simulink model "DroneModel"  (R2021b)
settings: Solver=VariableStepAuto  StartTime=0.0  StopTime=5  RelTol=1e-3
values from neighbouring files (symbols this model uses):
  g = 9.8    [testModel.m]
  Im = 0.0135^2*0.045/2    (= 4.100625e-06)    [testModel.m]
  Ip = (1.8*r)^2*0.015/12    (= 1.9845e-05)    [testModel.m]
  Ix = m/3*a^2/12+2*0.045*l^2    (= 0.00211347222222)    [testModel.m]
  Iy = m/3*a^2/12+4*0.045*l^2    (= 0.00413847222222)    [testModel.m]
  Iz = m/3*a^2/4+2*0.045*l^2    (= 0.00229041666667)    [testModel.m]
  J = 2.5*10^(-6)    (= 2.5e-06)    [testModel.m]
  Ke = ke    (= 0.0073)    [testModel.m]
  kf = ks*r^2*airDensity*Sblade/2    (= 1.57565625e-05)    [testModel.m]
  Km = kt    (= 0.0073)    [testModel.m]
  l = 0.15    [testModel.m]
  m = 0.65    [testModel.m]
  maxU = 11    [testModel.m]
  r = 0.07    [testModel.m]
  R = ra    (= 0.048)    [testModel.m]
  U1 = U1_arr(i)    [testModel.m]
  U2 = U2_arr(i)    [testModel.m]
  U3 = U3_arr(i)    [testModel.m]
  U4 = U4_arr(i)    [testModel.m]
settings Model: Creator=Degra  LastModifiedBy=Degra

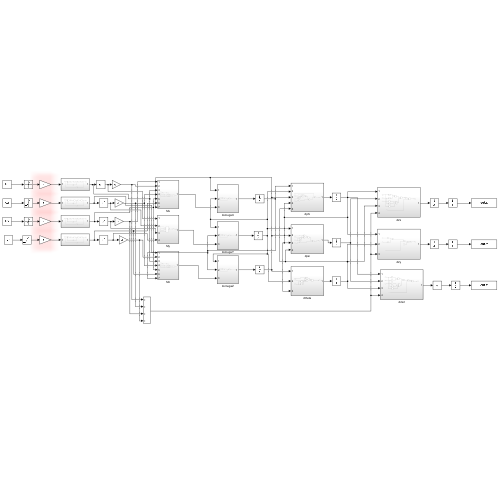
[thumbnail: Simulink's stored preview of the top-level diagram]
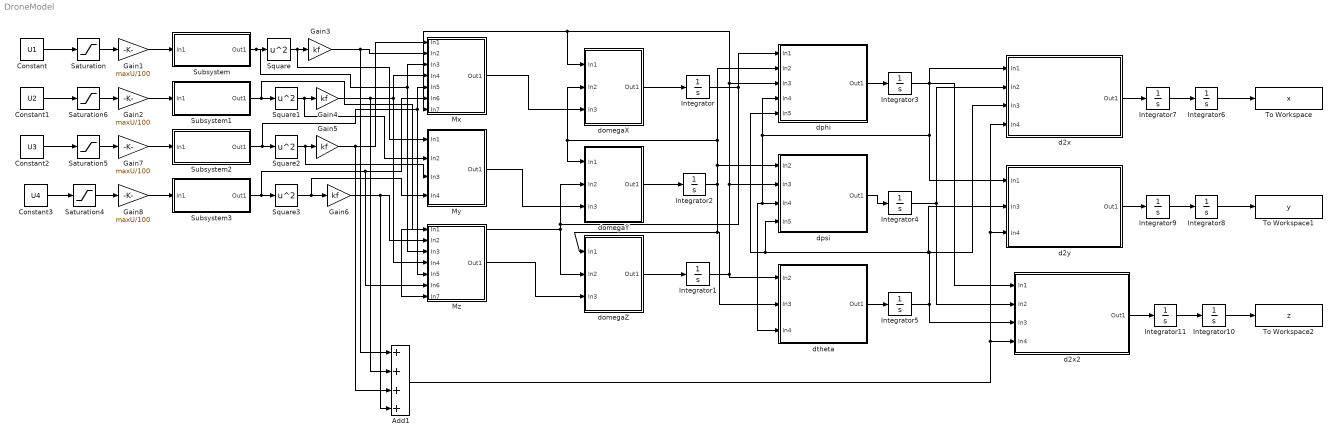
== system DroneModel ==
  Add1 : Sum  Inputs=++++
  Constant : Constant  Value=U1
  Constant1 : Constant  Value=U2
  Constant2 : Constant  Value=U3
  Constant3 : Constant  Value=U4
  Gain{1..2,7..8} (4 alike) : Gain  Gain=maxU/100
  Gain{3..6} (4 alike) : Gain  Gain=kf
  Integrator{,1..11} (12 alike) : Integrator
  Mx : Subsystem
  My : Subsystem
  Mz : Subsystem
  Saturation{,4..6} (4 alike) : Saturate  UpperLimit=100  LowerLimit=-100
  Square{,1..3} (4 alike) : Math  Operator=square  SaturateOnIntegerOverflow=on
  Subsystem : Subsystem
  Subsystem1 : Subsystem
  Subsystem2 : Subsystem
  Subsystem3 : Subsystem
  To Workspace : ToWorkspace  VariableName=x  SaveFormat=Timeseries  SampleTime=-1
  To Workspace1 : ToWorkspace  VariableName=y  SaveFormat=Timeseries  SampleTime=-1
  To Workspace2 : ToWorkspace  VariableName=z  SaveFormat=Timeseries  SampleTime=-1
  d2x : Subsystem
  d2x2 : Subsystem
  d2y : Subsystem
  domegaX : Subsystem
  domegaY : Subsystem
  domegaZ : Subsystem
  dphi : Subsystem
  dpsi : Subsystem
  dtheta : Subsystem
  wires:
  Subsystem/1(Out1) -> Mz/3(In3), Mx/3(In3), Square/1
  Square/1 -> My/1(In1), Gain3/1
  Subsystem1/1(Out1) -> Add1/2, Mz/4(In4), Mx/4(In4), Square1/1
  Square1/1 -> My/2(In2), Gain4/1
  Square2/1 -> My/3(In3), Gain5/1
  Subsystem3/1(Out1) -> Mz/6(In6), Mx/6(In6), Square3/1
  Square3/1 -> My/4(In4), Gain6/1
  Gain5/1 -> Add1/3, Mx/1(In1)
  Gain3/1 -> Add1/1, Mx/2(In2)
  Gain4/1 -> Mz/1(In1)
  Gain6/1 -> Add1/4, Mz/2(In2)
  Subsystem2/1(Out1) -> Mz/5(In5), Mx/5(In5), Square2/1
  Mx/1(Out1) -> domegaX/3(In3)
  domegaX/1(Out1) -> Integrator/1
  Integrator/1 -> domegaZ/2(In2), Mz/7(In7), domegaY/2(In2), dphi/1(In1)
  domegaZ/1(Out1) -> Integrator1/1
  Integrator1/1 -> dtheta/1(In2), dphi/3(In3), domegaX/1(In1), Mx/7(In7), dpsi/2(In3)
  Mz/1(Out1) -> domegaZ/3(In3)
  My/1(Out1) -> domegaY/3(In3)
  domegaY/1(Out1) -> Integrator2/1
  Integrator2/1 -> dphi/2(In2), domegaY/1(In1), domegaX/2(In2), dpsi/1(In2), domegaZ/1(In1), dtheta/2(In3)
  dpsi/1(Out1) -> Integrator4/1
  dphi/1(Out1) -> Integrator3/1
  Integrator3/1 -> d2x2/1(In1), d2x/1(In1), d2y/1(In1), dtheta/3(In4), dpsi/3(In4), dphi/4(In4)
  dtheta/1(Out1) -> Integrator5/1
  Integrator5/1 -> d2x2/3(In3), d2x/3(In3), d2y/2(In3), dpsi/4(In5), dphi/5(In5)
  Integrator4/1 -> d2x2/2(In2), d2x/2(In2)
  Add1/1 -> d2x2/4(In4), d2y/3(In4), d2x/4(In4)
  d2x/1(Out1) -> Integrator7/1
  Integrator7/1 -> Integrator6/1
  Integrator9/1 -> Integrator8/1
  d2y/1(Out1) -> Integrator9/1
  Integrator11/1 -> Integrator10/1
  d2x2/1(Out1) -> Integrator11/1
  Integrator6/1 -> To Workspace/1
  Integrator8/1 -> To Workspace1/1
  Integrator10/1 -> To Workspace2/1
  Constant/1 -> Saturation/1
  Constant3/1 -> Saturation4/1
  Constant2/1 -> Saturation5/1
  Constant1/1 -> Saturation6/1
  Saturation/1 -> Gain1/1
  Saturation6/1 -> Gain2/1
  Saturation4/1 -> Gain8/1
  Gain1/1 -> Subsystem/1(In1)
  Gain8/1 -> Subsystem3/1(In1)
  Gain7/1 -> Subsystem2/1(In1)
  Gain2/1 -> Subsystem1/1(In1)
  Saturation5/1 -> Gain7/1

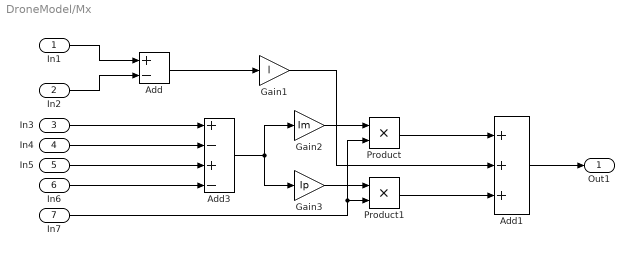
== system DroneModel/Mx ==
  In1 : Inport
  In2 : Inport  Port=2
  In3 : Inport  Port=3
  In4 : Inport  Port=4
  In5 : Inport  Port=5
  In6 : Inport  Port=6
  In7 : Inport  Port=7
  Add : Sum  Inputs=+-
  Add1 : Sum  Inputs=+++
  Add3 : Sum  Inputs=+-+-
  Gain1 : Gain  Gain=l
  Gain2 : Gain  Gain=Im
  Gain3 : Gain  Gain=Ip
  Product : Product
  Product1 : Product
  Out1 : Outport
  wires:
  In1/1 -> Add/1
  In2/1 -> Add/2
  In3/1 -> Add3/1
  In4/1 -> Add3/2
  In5/1 -> Add3/3
  In6/1 -> Add3/4
  Add/1 -> Gain1/1
  Add3/1 -> Gain3/1, Gain2/1
  Gain3/1 -> Product1/1
  Gain2/1 -> Product/1
  In7/1 -> Product1/2, Product/2
  Product1/1 -> Add1/3
  Product/1 -> Add1/1
  Gain1/1 -> Add1/2
  Add1/1 -> Out1/1

== system DroneModel/My ==
  In1 : Inport
  In2 : Inport  Port=2
  In3 : Inport  Port=3
  In4 : Inport  Port=4
  Add3 : Sum  Inputs=-+-+
  Gain3 : Gain  Gain=kf*r
  Out1 : Outport
  wires:
  Add3/1 -> Gain3/1
  In1/1 -> Add3/1
  In2/1 -> Add3/2
  In3/1 -> Add3/3
  In4/1 -> Add3/4
  Gain3/1 -> Out1/1

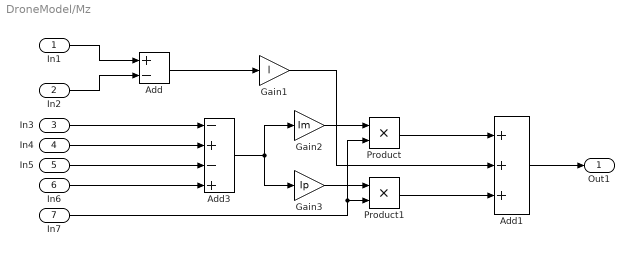
== system DroneModel/Mz ==
  In1 : Inport
  In2 : Inport  Port=2
  In3 : Inport  Port=3
  In4 : Inport  Port=4
  In5 : Inport  Port=5
  In6 : Inport  Port=6
  In7 : Inport  Port=7
  Add : Sum  Inputs=+-
  Add1 : Sum  Inputs=+++
  Add3 : Sum  Inputs=-+-+
  Gain1 : Gain  Gain=l
  Gain2 : Gain  Gain=Im
  Gain3 : Gain  Gain=Ip
  Product : Product
  Product1 : Product
  Out1 : Outport
  wires:
  In1/1 -> Add/1
  In2/1 -> Add/2
  In3/1 -> Add3/1
  In4/1 -> Add3/2
  In5/1 -> Add3/3
  In6/1 -> Add3/4
  Add/1 -> Gain1/1
  Add3/1 -> Gain3/1, Gain2/1
  Gain3/1 -> Product1/1
  Gain2/1 -> Product/1
  In7/1 -> Product1/2, Product/2
  Product1/1 -> Add1/3
  Product/1 -> Add1/1
  Gain1/1 -> Add1/2
  Add1/1 -> Out1/1

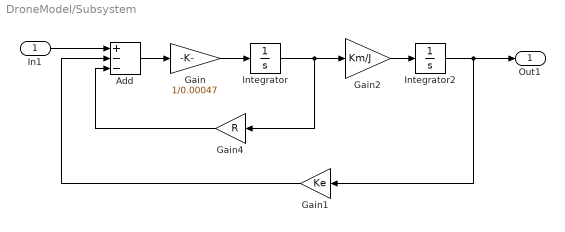
== system DroneModel/Subsystem ==
  In1 : Inport
  Add : Sum  Inputs=+--
  Gain : Gain  Gain=1/0.00047
  Gain1 : Gain  Gain=Ke
  Gain2 : Gain  Gain=Km/J
  Gain4 : Gain  Gain=R
  Integrator : Integrator
  Integrator2 : Integrator
  Out1 : Outport
  wires:
  In1/1 -> Add/1
  Gain4/1 -> Add/3
  Gain1/1 -> Add/2
  Integrator2/1 -> Out1/1, Gain1/1
  Integrator/1 -> Gain2/1, Gain4/1
  Gain2/1 -> Integrator2/1
  Add/1 -> Gain/1
  Gain/1 -> Integrator/1

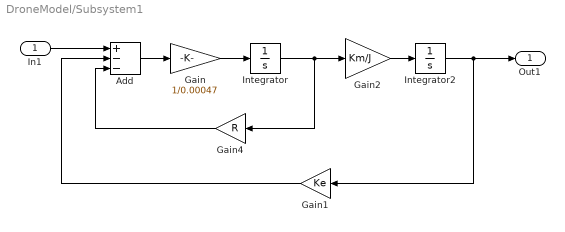
== system DroneModel/Subsystem1 ==
  In1 : Inport
  Add : Sum  Inputs=+--
  Gain : Gain  Gain=1/0.00047
  Gain1 : Gain  Gain=Ke
  Gain2 : Gain  Gain=Km/J
  Gain4 : Gain  Gain=R
  Integrator : Integrator
  Integrator2 : Integrator
  Out1 : Outport
  wires:
  In1/1 -> Add/1
  Gain4/1 -> Add/3
  Gain1/1 -> Add/2
  Integrator2/1 -> Out1/1, Gain1/1
  Integrator/1 -> Gain2/1, Gain4/1
  Gain2/1 -> Integrator2/1
  Add/1 -> Gain/1
  Gain/1 -> Integrator/1

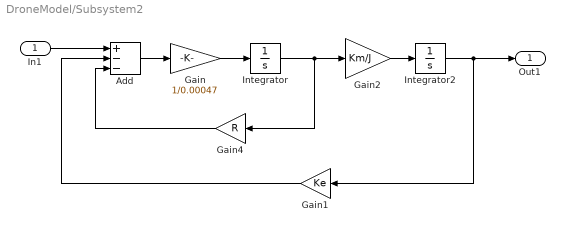
== system DroneModel/Subsystem2 ==
  In1 : Inport
  Add : Sum  Inputs=+--
  Gain : Gain  Gain=1/0.00047
  Gain1 : Gain  Gain=Ke
  Gain2 : Gain  Gain=Km/J
  Gain4 : Gain  Gain=R
  Integrator : Integrator
  Integrator2 : Integrator
  Out1 : Outport
  wires:
  In1/1 -> Add/1
  Gain4/1 -> Add/3
  Gain1/1 -> Add/2
  Integrator2/1 -> Out1/1, Gain1/1
  Integrator/1 -> Gain2/1, Gain4/1
  Gain2/1 -> Integrator2/1
  Add/1 -> Gain/1
  Gain/1 -> Integrator/1

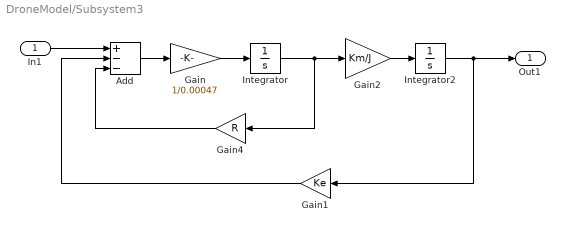
== system DroneModel/Subsystem3 ==
  In1 : Inport
  Add : Sum  Inputs=+--
  Gain : Gain  Gain=1/0.00047
  Gain1 : Gain  Gain=Ke
  Gain2 : Gain  Gain=Km/J
  Gain4 : Gain  Gain=R
  Integrator : Integrator
  Integrator2 : Integrator
  Out1 : Outport
  wires:
  In1/1 -> Add/1
  Gain4/1 -> Add/3
  Gain1/1 -> Add/2
  Integrator2/1 -> Out1/1, Gain1/1
  Integrator/1 -> Gain2/1, Gain4/1
  Gain2/1 -> Integrator2/1
  Add/1 -> Gain/1
  Gain/1 -> Integrator/1

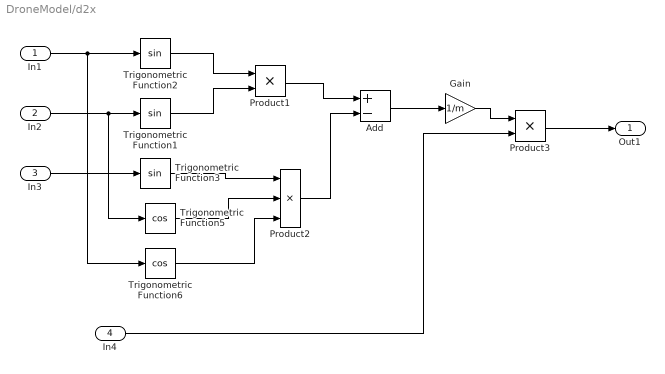
== system DroneModel/d2x ==
  In1 : Inport
  In2 : Inport  Port=2
  In3 : Inport  Port=3
  In4 : Inport  Port=4
  Add : Sum  Inputs=+-
  Gain : Gain  Gain=1/m
  Product1 : Product
  Product2 : Product  Inputs=3
  Product3 : Product
  Trigonometric Function1 : Trigonometry
  Trigonometric Function2 : Trigonometry
  Trigonometric Function3 : Trigonometry
  Trigonometric Function5 : Trigonometry  Operator=cos
  Trigonometric Function6 : Trigonometry  Operator=cos
  Out1 : Outport
  wires:
  In1/1 -> Trigonometric Function6/1, Trigonometric Function2/1
  In2/1 -> Trigonometric Function5/1, Trigonometric Function1/1
  Trigonometric Function2/1 -> Product1/1
  Trigonometric Function1/1 -> Product1/2
  Product1/1 -> Add/1
  In3/1 -> Trigonometric Function3/1
  Trigonometric Function3/1 -> Product2/1
  Trigonometric Function5/1 -> Product2/2
  Trigonometric Function6/1 -> Product2/3
  Product2/1 -> Add/2
  Add/1 -> Gain/1
  Gain/1 -> Product3/1
  In4/1 -> Product3/2
  Product3/1 -> Out1/1

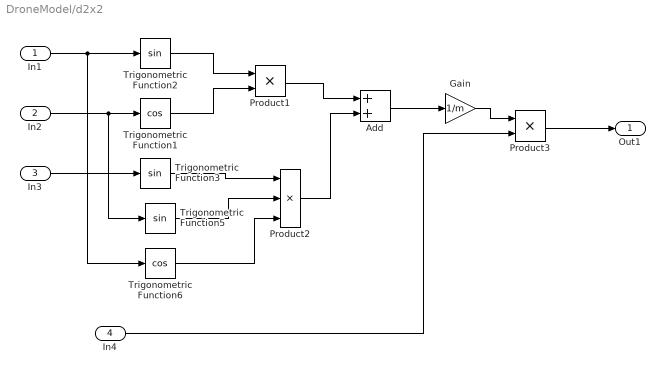
== system DroneModel/d2x2 ==
  In1 : Inport
  In2 : Inport  Port=2
  In3 : Inport  Port=3
  In4 : Inport  Port=4
  Add : Sum
  Gain : Gain  Gain=1/m
  Product1 : Product
  Product2 : Product  Inputs=3
  Product3 : Product
  Trigonometric Function1 : Trigonometry  Operator=cos
  Trigonometric Function2 : Trigonometry
  Trigonometric Function3 : Trigonometry
  Trigonometric Function5 : Trigonometry
  Trigonometric Function6 : Trigonometry  Operator=cos
  Out1 : Outport
  wires:
  In1/1 -> Trigonometric Function6/1, Trigonometric Function2/1
  In2/1 -> Trigonometric Function5/1, Trigonometric Function1/1
  Product1/1 -> Add/1
  In3/1 -> Trigonometric Function3/1
  Product2/1 -> Add/2
  Add/1 -> Gain/1
  Gain/1 -> Product3/1
  In4/1 -> Product3/2
  Product3/1 -> Out1/1
  Trigonometric Function1/1 -> Product1/2
  Trigonometric Function2/1 -> Product1/1
  Trigonometric Function3/1 -> Product2/1
  Trigonometric Function5/1 -> Product2/2
  Trigonometric Function6/1 -> Product2/3

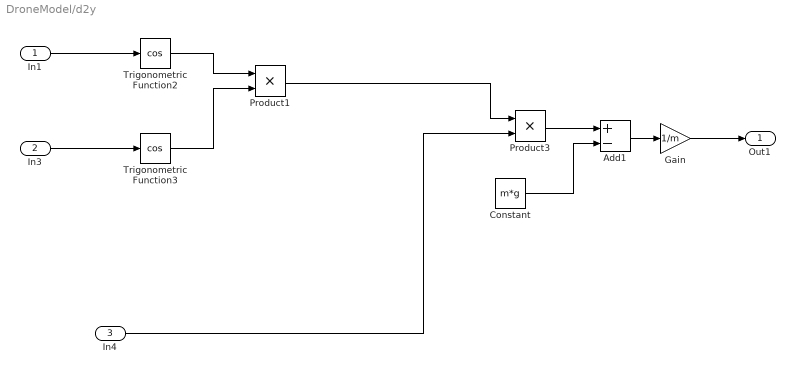
== system DroneModel/d2y ==
  In1 : Inport
  In3 : Inport  Port=2
  In4 : Inport  Port=3
  Add1 : Sum  Inputs=+-
  Constant : Constant  Value=m*g
  Gain : Gain  Gain=1/m
  Product1 : Product
  Product3 : Product
  Trigonometric Function2 : Trigonometry  Operator=cos
  Trigonometric Function3 : Trigonometry  Operator=cos
  Out1 : Outport
  wires:
  In1/1 -> Trigonometric Function2/1
  Trigonometric Function2/1 -> Product1/1
  In3/1 -> Trigonometric Function3/1
  Product1/1 -> Product3/1
  In4/1 -> Product3/2
  Product3/1 -> Add1/1
  Constant/1 -> Add1/2
  Add1/1 -> Gain/1
  Gain/1 -> Out1/1
  Trigonometric Function3/1 -> Product1/2

== system DroneModel/domegaX ==
  In1 : Inport
  In2 : Inport  Port=2
  In3 : Inport  Port=3
  Add : Sum
  Gain1 : Gain  Gain=(Iy-Iz)
  Gain2 : Gain  Gain=1/Ix
  Product : Product
  Out1 : Outport
  wires:
  In1/1 -> Product/1
  In2/1 -> Product/2
  In3/1 -> Add/2
  Product/1 -> Gain1/1
  Gain2/1 -> Out1/1
  Gain1/1 -> Add/1
  Add/1 -> Gain2/1

== system DroneModel/domegaY ==
  In1 : Inport
  In2 : Inport  Port=2
  In3 : Inport  Port=3
  Add : Sum
  Gain1 : Gain  Gain=(Iz-Ix)
  Gain2 : Gain  Gain=1/Iy
  Product : Product
  Out1 : Outport
  wires:
  In1/1 -> Product/1
  In2/1 -> Product/2
  In3/1 -> Add/2
  Product/1 -> Gain1/1
  Gain2/1 -> Out1/1
  Gain1/1 -> Add/1
  Add/1 -> Gain2/1

== system DroneModel/domegaZ ==
  In1 : Inport
  In2 : Inport  Port=2
  In3 : Inport  Port=3
  Add : Sum
  Gain1 : Gain  Gain=(Ix-Iy)
  Gain2 : Gain  Gain=1/Iz
  Product : Product
  Out1 : Outport
  wires:
  In1/1 -> Product/1
  In2/1 -> Product/2
  In3/1 -> Add/2
  Product/1 -> Gain1/1
  Gain2/1 -> Out1/1
  Gain1/1 -> Add/1
  Add/1 -> Gain2/1

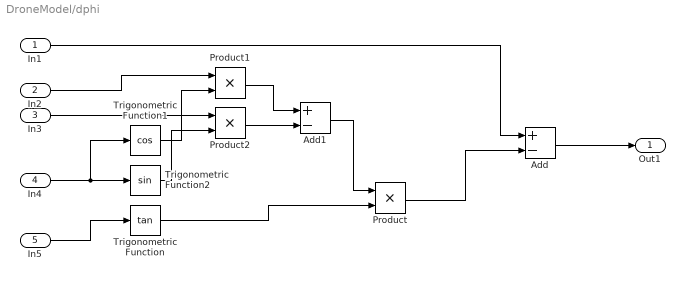
== system DroneModel/dphi ==
  In1 : Inport
  In2 : Inport  Port=2
  In3 : Inport  Port=3
  In4 : Inport  Port=4
  In5 : Inport  Port=5
  Add : Sum  Inputs=+-
  Add1 : Sum  Inputs=+-
  Product : Product
  Product1 : Product
  Product2 : Product
  Trigonometric Function : Trigonometry  Operator=tan
  Trigonometric Function1 : Trigonometry  Operator=cos
  Trigonometric Function2 : Trigonometry
  Out1 : Outport
  wires:
  Trigonometric Function/1 -> Product/2
  Trigonometric Function1/1 -> Product1/2
  In5/1 -> Trigonometric Function/1
  In1/1 -> Add/1
  In2/1 -> Product1/1
  In3/1 -> Product2/1
  In4/1 -> Trigonometric Function2/1, Trigonometric Function1/1
  Product1/1 -> Add1/1
  Product2/1 -> Add1/2
  Trigonometric Function2/1 -> Product2/2
  Add/1 -> Out1/1
  Add1/1 -> Product/1
  Product/1 -> Add/2

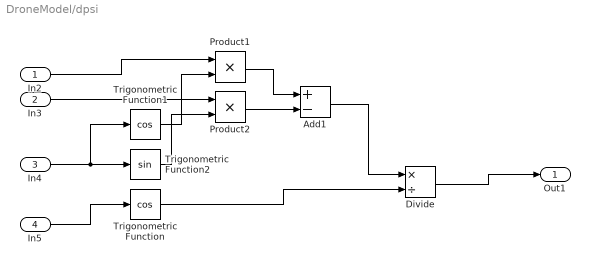
== system DroneModel/dpsi ==
  In2 : Inport
  In3 : Inport  Port=2
  In4 : Inport  Port=3
  In5 : Inport  Port=4
  Add1 : Sum  Inputs=+-
  Divide : Product  Inputs=*/
  Product1 : Product
  Product2 : Product
  Trigonometric Function : Trigonometry  Operator=cos
  Trigonometric Function1 : Trigonometry  Operator=cos
  Trigonometric Function2 : Trigonometry
  Out1 : Outport
  wires:
  Trigonometric Function/1 -> Divide/2
  Trigonometric Function1/1 -> Product1/2
  In5/1 -> Trigonometric Function/1
  In2/1 -> Product1/1
  In3/1 -> Product2/1
  In4/1 -> Trigonometric Function2/1, Trigonometric Function1/1
  Product1/1 -> Add1/1
  Product2/1 -> Add1/2
  Trigonometric Function2/1 -> Product2/2
  Divide/1 -> Out1/1
  Add1/1 -> Divide/1

== system DroneModel/dtheta ==
  In2 : Inport
  In3 : Inport  Port=2
  In4 : Inport  Port=3
  Add1 : Sum
  Product1 : Product
  Product2 : Product
  Trigonometric Function1 : Trigonometry  Operator=cos
  Trigonometric Function2 : Trigonometry
  Out1 : Outport
  wires:
  Trigonometric Function1/1 -> Product1/2
  In2/1 -> Product1/1
  In3/1 -> Product2/1
  In4/1 -> Trigonometric Function2/1, Trigonometric Function1/1
  Product1/1 -> Add1/1
  Product2/1 -> Add1/2
  Trigonometric Function2/1 -> Product2/2
  Add1/1 -> Out1/1
